simulink model "c10mpopt"  (R2021b)
settings: Solver=VariableStepAuto  StartTime=0.0  StopTime=20  RelTol=1e-3  EnableMultiTasking=on
undefined symbols (not defined in the file): G, u1, u2
libraries: cstblocks x2
settings Model: Creator=Dingyu  LastModifiedBy=xuedi
settings SolverCC: AlgebraicLoopSolver=TrustRegion
settings DataIOCC: ReturnWorkspaceOutputs=off
settings OptimizationCC: LifeSpan=inf
settings DebuggingCC: SFUnexpectedBacktrackingDiag=warning  SFNoUnconditionalDefaultTransitionDiag=warning  SFMachineParentedDataDiag=warning  ArithmeticOperatorsInVariantConditions=warning
settings SFSimCC: SimUseLocalCustomCode=off  CustomCodeUndefinedFunction=UseInterfaceOnly
settings RTWCC: RTWUseLocalCustomCode=off
settings CodeAppCC: StateflowObjectComments=on
settings GRTTargetCC: TargetLangStandard=C89/C90 (ANSI)
settings ConfigComp: CovMetricSettings=dw  CovSaveCumulativeToWorkspaceVar=on  CovSaveSingleToWorkspaceVar=on  CovExternalEMLEnable=off

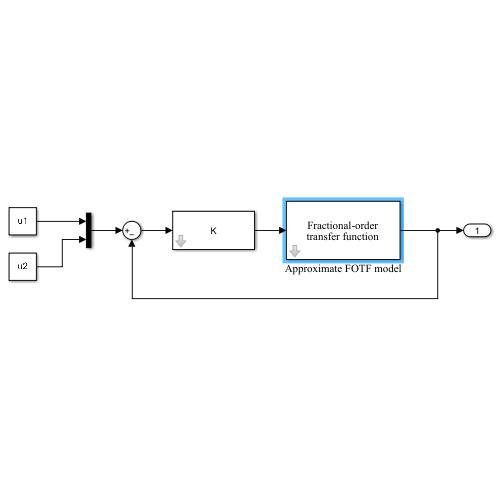
[thumbnail: Simulink's stored preview of the top-level diagram]
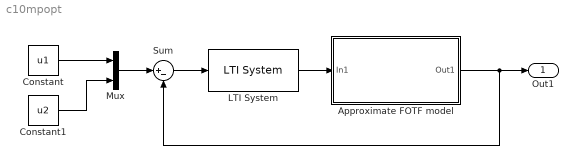
== system c10mpopt ==
  Approximate FOTF model : Subsystem  mask{na=G, a=[1 3.3 2.9 3.32 1], nb=0, b=1, N=9, ww=[1e-5 1e3], kF=Oustaloup filter, T=0}
      mask prompts: na "Orders of the denominator"; a "Coefficients of the denominator"; nb "Orders of the numerator"; b "Coefficients of the numerator"; N "Filter order"; ww "Interested frequency range [wb wh]"; kF "Types of the filter"; T "Delay constant T"
      mask init:
      | if isa(na,'fotf'), G=na; T=G.ioDelay;
      | else
      |     if length(na)~=length(a), errordlg('Error','Mismatch on the denominator'), end
      |     if length(b)~=length(nb), errordlg('Error','Mismatch on the denominator'), end
      |     G=fotf(a,na,b,nb,T); 
      | end
      | if kF==1, str='ousta_fod'; else, str='new_fod'; end
      | wb=ww(1); wh=ww(2);
      | G1=high_order(G,str,wb,wh,N); G1.ioDelay=T;
      mask TypeOptions kF: Oustaloup filter | Modified Oustaloup filter
      mask Display: disp('Fractional-order\ntransfer function')
  Constant : Constant  Value=u1
  Constant1 : Constant  Value=u2
  LTI System : cstblocks/LTI System  sys=K  IC=[]
  Mux : Mux  Inputs=2
  Sum : Sum  Inputs=|+-
  Out1 : Outport
  wires:
  Sum/1 -> LTI System/1
  Mux/1 -> Sum/1
  Constant/1 -> Mux/1
  Constant1/1 -> Mux/2
  LTI System/1 -> Approximate FOTF model/1(In1)
  Approximate FOTF model/1(Out1) -> Sum/2, Out1/1

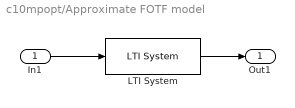
== system c10mpopt/Approximate FOTF model ==
  In1 : Inport
  LTI System : cstblocks/LTI System  sys=G1  IC=[]
  Out1 : Outport
  wires:
  In1/1 -> LTI System/1
  LTI System/1 -> Out1/1
